simulink library "amg_high_precision_rtc"  (R2015b)
settings: Solver=ode45  StartTime=0.0  StopTime=10.0  RelTol=1e-3
libraries: simulink x207, waijung_soft_i2c_lib x11, amg_high_precision_rtc x10
(part 1 of 5)
settings Model: Creator=Krisada  LastModifiedBy=Aimagin
settings DataIOCC: SaveFormat=Array  SignalLoggingSaveFormat=ModelDataLogs
settings OptimizationCC: BlockReduction=off  DefaultParameterBehavior=Inlined  BufferReuse=off  ExpressionDepthLimit=2147483647
settings DebuggingCC: UnderspecifiedInitializationDetection=Classic  MergeDetectMultiDrivingBlocksExec=none  SolverPrmCheckMsg=warning  FcnCallInpInsideContextMsg=UseLocalSettings  StateNameClashWarn=warning  StrictBusMsg=Warning
settings HardwareCC: ProdBitPerPointer=32  ProdLargestAtomicFloat=None  ProdIntDivRoundTo=Undefined  ProdEndianess=Unspecified  ProdWordSize=32  ProdHWDeviceType=32-bit Generic
settings GRTTargetCC: CombineOutputUpdateFcns=off  GRTInterface=on
settings ConfigComp: CovModelRefEnable=Off

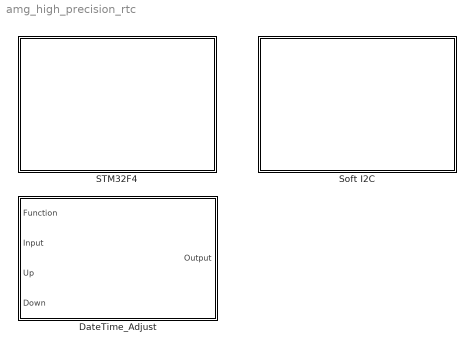
== system amg_high_precision_rtc ==
  DateTime_Adjust : Subsystem  TreatAsAtomicUnit=on  mask{state=0, max=99, min=0}
      mask prompts: state "Adjust state"; max "Max limit"; min "Min limit"
      settings: RTWFcnNameOpts=Use subsystem name  RTWFileNameOpts=Use function name
  STM32F4 : Subsystem
  Soft I2C : Subsystem

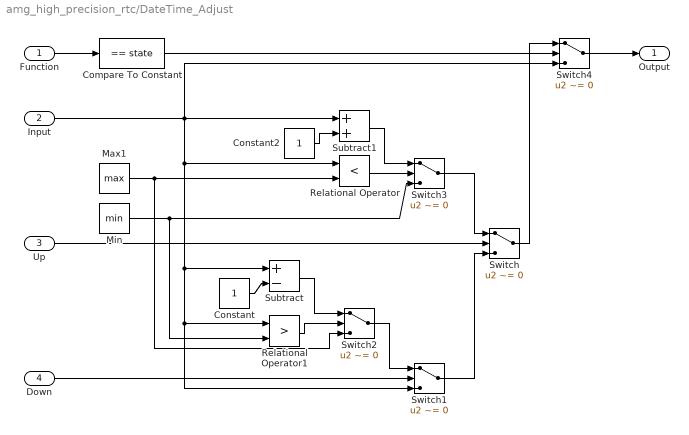
== system amg_high_precision_rtc/DateTime_Adjust ==
  Function : Inport
  Input : Inport  Port=2
  Up : Inport  Port=3
  Down : Inport  Port=4
  Compare To Constant : simulink/Logic and Bit Operations/Compare To Constant  SystemSampleTime=-1  relop===  const=state  LogicOutDataTypeMode=uint8  ZeroCross=off
  Constant : Constant  OutDataTypeStr=uint8
  Constant2 : Constant  OutDataTypeStr=uint8
  Max1 : Constant  Value=max  OutDataTypeStr=uint8
  Min : Constant  Value=min  OutDataTypeStr=uint8
  Relational Operator : RelationalOperator  Operator=<  OutDataTypeStr=boolean
  Relational Operator1 : RelationalOperator  Operator=>  OutDataTypeStr=boolean
  Subtract : Sum  Inputs=+-
  Subtract1 : Sum
  Switch{,1..4} (5 alike) : Switch  Criteria=u2 ~= 0
  Output : Outport
  wires:
  Switch1/1 -> Switch/3
  Input/1 -> Subtract/1, Switch1/3, Relational Operator1/1, Relational Operator/1, Subtract1/1, Switch4/3
  Relational Operator1/1 -> Switch2/2
  Subtract/1 -> Switch2/1
  Constant/1 -> Subtract/2
  Switch2/1 -> Switch1/1
  Relational Operator/1 -> Switch3/2
  Subtract1/1 -> Switch3/1
  Constant2/1 -> Subtract1/2
  Min/1 -> Switch3/3, Relational Operator1/2
  Max1/1 -> Relational Operator/2, Switch2/3
  Switch3/1 -> Switch/1
  Function/1 -> Compare To Constant/1
  Switch4/1 -> Output/1
  Compare To Constant/1 -> Switch4/2
  Switch/1 -> Switch4/1
  Down/1 -> Switch1/2
  Up/1 -> Switch/2

== system amg_high_precision_rtc/STM32F4 ==
  DS3231 Configure : Subsystem  mask(amg_high_precision_rtc){blockfunction=configure, module=1}
      mask prompts: blockfunction "Function"; module "I2C module"
      mask init:
      | amg_high_precision_rtc_callback('init');
      mask Help: web(fullfile(waijungdocroot,'DS3231_Configure.htm'), '-browser')
      mask TypeOptions blockfunction: temp | time | date | configure
      mask TypeOptions module: 1 | 2 | 3
      mask Callback module: amg_high_precision_rtc_callback('module');
      mask Display: text(0.5, 0.5, 'Port: I2C1','ver','middle','hor','center');port_label('input', 1,'SlvAddr');port_label('output', 1,'Status');port_label('input', 2,'(+) UP');port_label('input', 3,'(-) DOWN');port_label('input', 4,'(*) MODE');port_label('output', 2,'Enable');
  DS3231 Get Date : Subsystem  mask(amg_high_precision_rtc){blockfunction=date, module=1}
      mask prompts: blockfunction "Function"; module "I2C module"
      mask init:
      | amg_high_precision_rtc_callback('init');
      mask Help: web(fullfile(waijungdocroot,'DS3231_Get_Date.htm'), '-browser')
      mask TypeOptions blockfunction: temp | time | date
      mask TypeOptions module: 1 | 2 | 3
      mask Callback module: amg_high_precision_rtc_callback('module');
      mask Display: text(0.5, 0.5, 'Port: I2C1','ver','middle','hor','center');port_label('input', 1,'SlvAddr');port_label('output', 1,'Status');port_label('output', 2,'Day(1-7)');port_label('output', 3,'Date(1-31)');port_label('output', 4,'Month(1-12)');port_label('output', 5,'Year(0-99)');
  DS3231 Get Time : Subsystem  mask(amg_high_precision_rtc){blockfunction=time, module=1}
      mask prompts: blockfunction "Function"; module "I2C module"
      mask init:
      | amg_high_precision_rtc_callback('init');
      mask Help: web(fullfile(waijungdocroot,'DS3231_Get_Time.htm'), '-browser')
      mask TypeOptions blockfunction: temp | time | date
      mask TypeOptions module: 1 | 2 | 3
      mask Callback module: amg_high_precision_rtc_callback('module');
      mask Display: text(0.5, 0.5, 'Port: I2C1','ver','middle','hor','center');port_label('input', 1,'SlvAddr');port_label('output', 1,'Status');port_label('output', 2,'Hour(0-11/23)');port_label('output', 3,'Minute(0-59)');port_label('output', 4,'Second(0-59)');port_label('output', 5,'AM(0)/PM(1)');
  DS3231 Set Date : Subsystem  mask(amg_high_precision_rtc){blockfunction=setdate, module=1}
      mask prompts: blockfunction "Function"; module "I2C module"
      mask init:
      | amg_high_precision_rtc_callback('init');
      mask Help: web(fullfile(waijungdocroot,'DS3231_Get_Time.htm'), '-browser')
      mask TypeOptions blockfunction: setdate
      mask TypeOptions module: 1 | 2 | 3
      mask Callback module: amg_high_precision_rtc_callback('module');
      mask Display: text(0.5, 0.5, 'Port: I2C1','ver','middle','hor','center');port_label('input', 1,'SlvAddr');port_label('input', 2,'Date(1-31)');port_label('input', 3,'Month(1-12)');port_label('input', 4,'Year(0-99)');port_label('output', 1,'Status');
  DS3231 Set Time : Subsystem  mask(amg_high_precision_rtc){blockfunction=settime, module=1}
      mask prompts: blockfunction "Function"; module "I2C module"
      mask init:
      | amg_high_precision_rtc_callback('init');
      mask Help: web(fullfile(waijungdocroot,'DS3231_Get_Date.htm'), '-browser')
      mask TypeOptions blockfunction: settime
      mask TypeOptions module: 1 | 2 | 3
      mask Callback module: amg_high_precision_rtc_callback('module');
      mask Display: text(0.5, 0.5, 'Port: I2C1','ver','middle','hor','center');port_label('input', 1,'SlvAddr');port_label('input', 2,'Hour(0-11/23)');port_label('input', 3,'Minute(0-59)');port_label('input', 4,'Second(0-59)');port_label('output', 1,'Status');
  DS3231Temperture : Subsystem  mask(amg_high_precision_rtc){blockfunction=temp, module=1}
      mask prompts: blockfunction "Function"; module "I2C module"
      mask help:
      | The block implement temperature reading from DS3231 (Extremely Accurate RTC).
      | Its override the CONV bit, to force the temperature update, so the recommend sample time for this block is more than 0.5 seconds.
      | To get reading value from DS3231 device, this block generate 3 transaction of I2C as below:
      | 1. Read 2 bytes data from register 0x11 and 0x12 (Sequential read).
      | 2. Read 1 byte data from register 0x0F (Status) for poll BSY bit.
      | 3. Write 1 byte data to register 0x0E to force temperature conversion, CONV bit.
      mask init:
      | amg_high_precision_rtc_callback('init');
      mask Help: web(fullfile(waijungdocroot,'DS3231Temperture.htm'), '-browser')
      mask TypeOptions blockfunction: temp | time | date
      mask TypeOptions module: 1 | 2 | 3
      mask Callback module: amg_high_precision_rtc_callback('module');
      mask Display: text(0.5, 0.5, 'Port: I2C1','ver','middle','hor','center');port_label('input', 1,'SlvAddr');port_label('output', 1,'Status');port_label('output', 2,'Temp (C)');

== system amg_high_precision_rtc/Soft I2C ==
  Soft-DS3231 Configure : Subsystem  mask(amg_high_precision_rtc){blockfunction=configure, module=1}
      mask prompts: blockfunction "Function"; module "I2C module"
      mask init:
      | amg_high_precision_rtc_callback('init');
      mask Help: web(fullfile(waijungdocroot,'DS3231_Configure.htm'), '-browser')
      mask TypeOptions blockfunction: temp | time | date | configure
      mask TypeOptions module: 1 | 2 | 3 | 4 | 5 | 6 | 7 | 8 | 9 | 10 | 11 | 12 | 13 | 14 | 15 | 16 | 17 | 18 | 19 | 20 | 21 | 22 | 23 | 24 | 25 | 26 | 27 | 28 | 29 | 30 | 31 | 32
      mask Callback module: amg_high_precision_rtc_callback('module');
      mask Display: text(0.5, 0.5, 'Port: I2C1','ver','middle','hor','center');port_label('input', 1,'SlvAddr');port_label('output', 1,'Status');port_label('input', 2,'(+) UP');port_label('input', 3,'(-) DOWN');port_label('input', 4,'(*) MODE');port_label('output', 2,'Enable');
  Soft-DS3231 Get Date : Subsystem  mask(amg_high_precision_rtc){blockfunction=date, module=1}
      mask prompts: blockfunction "Function"; module "I2C module"
      mask init:
      | amg_high_precision_rtc_callback('init');
      mask Help: web(fullfile(waijungdocroot,'DS3231_Get_Date.htm'), '-browser')
      mask TypeOptions blockfunction: temp | time | date
      mask TypeOptions module: 1 | 2 | 3 | 4 | 5 | 6 | 7 | 8 | 9 | 10 | 11 | 12 | 13 | 14 | 15 | 16 | 17 | 18 | 19 | 20 | 21 | 22 | 23 | 24 | 25 | 26 | 27 | 28 | 29 | 30 | 31 | 32
      mask Callback module: amg_high_precision_rtc_callback('module');
      mask Display: text(0.5, 0.5, 'Port: I2C1','ver','middle','hor','center');port_label('input', 1,'SlvAddr');port_label('output', 1,'Status');port_label('output', 2,'Day(1-7)');port_label('output', 3,'Date(1-31)');port_label('output', 4,'Month(1-12)');port_label('output', 5,'Year(0-99)');
  Soft-DS3231 Get Time : Subsystem  mask(amg_high_precision_rtc){blockfunction=time, module=1}
      mask prompts: blockfunction "Function"; module "I2C module"
      mask init:
      | amg_high_precision_rtc_callback('init');
      mask Help: web(fullfile(waijungdocroot,'DS3231_Get_Time.htm'), '-browser')
      mask TypeOptions blockfunction: temp | time | date
      mask TypeOptions module: 1 | 2 | 3 | 4 | 5 | 6 | 7 | 8 | 9 | 10 | 11 | 12 | 13 | 14 | 15 | 16 | 17 | 18 | 19 | 20 | 21 | 22 | 23 | 24 | 25 | 26 | 27 | 28 | 29 | 30 | 31 | 32
      mask Callback module: amg_high_precision_rtc_callback('module');
      mask Display: text(0.5, 0.5, 'Port: I2C1','ver','middle','hor','center');port_label('input', 1,'SlvAddr');port_label('output', 1,'Status');port_label('output', 2,'Hour(0-11/23)');port_label('output', 3,'Minute(0-59)');port_label('output', 4,'Second(0-59)');port_label('output', 5,'AM(0)/PM(1)');
  Soft-DS3231 Set Date : Subsystem  mask(amg_high_precision_rtc){blockfunction=setdate, module=1}
      mask prompts: blockfunction "Function"; module "I2C module"
      mask init:
      | amg_high_precision_rtc_callback('init');
      mask Help: web(fullfile(waijungdocroot,'DS3231_Get_Time.htm'), '-browser')
      mask TypeOptions blockfunction: setdate
      mask TypeOptions module: 1 | 2 | 3 | 4 | 5 | 6 | 7 | 8 | 9 | 10 | 11 | 12 | 13 | 14 | 15 | 16 | 17 | 18 | 19 | 20 | 21 | 22 | 23 | 24 | 25 | 26 | 27 | 28 | 29 | 30 | 31 | 32
      mask Callback module: amg_high_precision_rtc_callback('module');
      mask Display: text(0.5, 0.5, 'Port: I2C1','ver','middle','hor','center');port_label('input', 1,'SlvAddr');port_label('input', 2,'Date(1-31)');port_label('input', 3,'Month(1-12)');port_label('input', 4,'Year(0-99)');port_label('output', 1,'Status');
  Soft-DS3231 Set Time : Subsystem  mask(amg_high_precision_rtc){blockfunction=settime, module=1}
      mask prompts: blockfunction "Function"; module "I2C module"
      mask init:
      | amg_high_precision_rtc_callback('init');
      mask Help: web(fullfile(waijungdocroot,'DS3231_Get_Date.htm'), '-browser')
      mask TypeOptions blockfunction: settime
      mask TypeOptions module: 1 | 2 | 3 | 4 | 5 | 6 | 7 | 8 | 9 | 10 | 11 | 12 | 13 | 14 | 15 | 16 | 17 | 18 | 19 | 20 | 21 | 22 | 23 | 24 | 25 | 26 | 27 | 28 | 29 | 30 | 31 | 32
      mask Callback module: amg_high_precision_rtc_callback('module');
      mask Display: text(0.5, 0.5, 'Port: I2C1','ver','middle','hor','center');port_label('input', 1,'SlvAddr');port_label('input', 2,'Hour(0-11/23)');port_label('input', 3,'Minute(0-59)');port_label('input', 4,'Second(0-59)');port_label('output', 1,'Status');
  Soft-DS3231Temperture : Subsystem  mask(amg_high_precision_rtc){blockfunction=temp, module=1}
      mask prompts: blockfunction "Function"; module "I2C module"
      mask help:
      | The block implement temperature reading from DS3231 (Extremely Accurate RTC).
      | Its override the CONV bit, to force the temperature update, so the recommend sample time for this block is more than 0.5 seconds.
      | To get reading value from DS3231 device, this block generate 3 transaction of I2C as below:
      | 1. Read 2 bytes data from register 0x11 and 0x12 (Sequential read).
      | 2. Read 1 byte data from register 0x0F (Status) for poll BSY bit.
      | 3. Write 1 byte data to register 0x0E to force temperature conversion, CONV bit.
      mask init:
      | amg_high_precision_rtc_callback('init');
      mask Help: web(fullfile(waijungdocroot,'DS3231Temperture.htm'), '-browser')
      mask TypeOptions blockfunction: temp | time | date
      mask TypeOptions module: 1 | 2 | 3 | 4 | 5 | 6 | 7 | 8 | 9 | 10 | 11 | 12 | 13 | 14 | 15 | 16 | 17 | 18 | 19 | 20 | 21 | 22 | 23 | 24 | 25 | 26 | 27 | 28 | 29 | 30 | 31 | 32
      mask Callback module: amg_high_precision_rtc_callback('module');
      mask Display: text(0.5, 0.5, 'Port: I2C1','ver','middle','hor','center');port_label('input', 1,'SlvAddr');port_label('output', 1,'Status');port_label('output', 2,'Temp (C)');

== system amg_high_precision_rtc/STM32F4/DS3231 Configure ==
  Slave Address : Inport
  Button UP : Inport  Port=2
  Button DOWN : Inport  Port=3
  Button MODE : Inport  Port=4
  Debouce4 : Subsystem  TreatAsAtomicUnit=on  mask{mode=Toggle Latch, prescale=256, debouce=255}
      mask prompts: prescale "Prescale (Debouce count)"; debouce "Debouce value"
      settings: RTWFcnNameOpts=Use subsystem name  RTWFileNameOpts=Use function name
      mask TypeOptions mode: Normal | Single Pulse | Toggle Latch
      mask Callback mode: waijung_intput_validation_callback('mode');
      mask TypeOptions prescale: 4 | 8 | 16 | 32 | 64 | 128 | 256 | 512 | 1024 | 2048 | 4096 | 8192
      mask Callback debouce: waijung_intput_validation_callback('prescale');
      mask Display: disp('Button Pressed\n(Toggle Latch)\nDebounce count: 256');
  Enabled Subsystem : Subsystem  TreatAsAtomicUnit=on
  Adjust state : Outport
  Adjust enable : Outport  Port=2
  wires:
  Slave Address/1 -> Enabled Subsystem/1(SlvAddr)
  Button UP/1 -> Enabled Subsystem/2(UP)
  Button DOWN/1 -> Enabled Subsystem/3(DOWN)
  Button MODE/1 -> Debouce4/1(In1), Enabled Subsystem/4(MODE)
  Debouce4/1(Out1) -> Enabled Subsystem/Enable, Adjust enable/1
  Enabled Subsystem/1(Adjust state) -> Adjust state/1

== system amg_high_precision_rtc/STM32F4/DS3231 Get Date ==
  Slave Address : Inport
  Compare To Zero : simulink/Logic and Bit Operations/Compare To Zero  SystemSampleTime=-1  relop===  LogicOutDataTypeMode=uint8  ZeroCross=off
  Convert : Subsystem  TreatAsAtomicUnit=on
  I2C Master Read/Write : S-Function  FunctionName=stm32f4_i2c  Parameters=configuration,module,transfer,clkspeed,timeout,sdapin,sclpin,writecount,readcount,inputtypearray,outputtypearray,confstr,sampletime,sampletimestr,blockid  SFunctionDeploymentMode=off  EnableBusSupport=off  mask(stm32f4_i2c){configuration=Transaction, module=1, lastmodule=3, transfer=Blocking, dutycycle=TLow/THigh = 2, clkspeed=400, timeout=25, writecount=1, readcount=4, sdapin=C9, sclpin=A8, waitwritetime=0, inputtypearray=[2 3 3], outputtypearray=[5 3 3 3 3 3], confstr=["C","9","A","8","1","1","6","0","I2C_DutyCycle_2","0"], sampletime=-1, sampletimestr=0, blockid=amg_high_precision_rtcDS3231GetDateI2CMasterReadWrite}
      mask prompts: module "I2C Module"; lastmodule "Last module"; transfer "Transfer mode"; dutycycle "Duty cycle in fast mode"; clkspeed "Clock speed (kHz)"; timeout "Timeout (ms)"; writecount "Bytes write count"; readcount "Bytes read count"; sdapin "SDA pin"; sclpin "SCL pin"; waitwritetime "Wait write time (ms), default is 0"; inputtypearray "Input type array"; outputtypearray "Output type array"; confstr "Configuration string"; sampletime "Sample time (sec)"; sampletimestr "Compiled sample time (sec) in string"
      mask init:
      | stm32f4_i2c_callback('init');
      mask Help: web(fullfile(waijungdocroot,'stm32f4_i2c_readwrite.htm'), '-browser')
      mask TypeOptions configuration: Setup | Transaction
      mask Callback configuration: stm32f4_i2c_callback('configuration');
      mask TypeOptions module: 1 | 2 | 3
      mask Callback module: stm32f4_i2c_callback('module');
      mask TypeOptions transfer: Blocking | Non-blocking
      mask TypeOptions dutycycle: TLow/THigh = 16/9 | TLow/THigh = 2
      mask Callback dutycycle: stm32f4_i2c_callback('dutycycle');
      mask Callback writecount: stm32f4_i2c_callback('writecount');
      mask Callback readcount: stm32f4_i2c_callback('readcount');
      mask TypeOptions sdapin: - | C9
      mask Callback sdapin: stm32f4_i2c_callback('sdapin');
      mask TypeOptions sclpin: - | A8
      mask Callback sclpin: stm32f4_i2c_callback('sclpin');
      mask Callback confstr: stm32f4_i2c_callback('confstr');
      mask Callback sampletime: stm32f4_i2c_callback('sampletime');
      mask Callback sampletimestr: stm32f4_i2c_callback('sampletimestr');
      mask Callback blockid: stm32f4_i2c_callback('blockid');
      mask Display: text(0.5, 0.5, 'Module: I2C1\nTransfer: Blocking\nWrite: 1 bytes\nRead: 4 bytes\nTs (sec): 0','ver','middle','hor','center');port_label('input', 1,'SlvAddr');port_label('input', 2,'Wr0 (uint8)');port_label('output', 1,'Status');port_label('output', 2,'Rd0 (uint8)');port_label('output', 3,'Rd1 (uint8)');port_label('output', 4,'Rd2 (uint8)');port_label('output', 5,'Rd3 (uint8)');
  REG_DATE : Constant  Value=hex2dec('03')  OutDataTypeStr=uint8
  Status : Outport
  Day : Outport  Port=2
  Date : Outport  Port=3
  Month : Outport  Port=4
  Year : Outport  Port=5
  wires:
  I2C Master Read/Write/4 -> Convert/3(In3)
  I2C Master Read/Write/3 -> Convert/2(In2)
  I2C Master Read/Write/2 -> Convert/1(In1)
  Compare To Zero/1 -> Status/1, Convert/Enable
  I2C Master Read/Write/1 -> Compare To Zero/1
  Slave Address/1 -> I2C Master Read/Write/1
  REG_DATE/1 -> I2C Master Read/Write/2
  I2C Master Read/Write/5 -> Convert/4(In4)
  Convert/1(Day) -> Day/1
  Convert/2(Date) -> Date/1
  Convert/4(Year) -> Year/1
  Convert/3(Month) -> Month/1

== system amg_high_precision_rtc/STM32F4/DS3231 Get Time ==
  Slave Address : Inport
  Compare To Zero : simulink/Logic and Bit Operations/Compare To Zero  SystemSampleTime=-1  relop===  LogicOutDataTypeMode=uint8  ZeroCross=off
  Convert : Subsystem  TreatAsAtomicUnit=on
  Data Type Conversion{,1..3} (4 alike) : DataTypeConversion  OutDataTypeStr=uint8
  I2C Master Read/Write : S-Function  FunctionName=stm32f4_i2c  Parameters=configuration,module,transfer,clkspeed,timeout,sdapin,sclpin,writecount,readcount,inputtypearray,outputtypearray,confstr,sampletime,sampletimestr,blockid  SFunctionDeploymentMode=off  EnableBusSupport=off  mask(stm32f4_i2c){configuration=Transaction, module=1, lastmodule=3, transfer=Blocking, dutycycle=TLow/THigh = 2, clkspeed=400, timeout=25, writecount=1, readcount=3, sdapin=C9, sclpin=A8, waitwritetime=0, inputtypearray=[2 3 3], outputtypearray=[4 3 3 3 3], confstr=["C","9","A","8","1","1","6","0","I2C_DutyCycle_2","0"], sampletime=-1, sampletimestr=0, blockid=amg_high_precision_rtcDS3231TimeI2CMasterReadWrite}
      mask prompts: module "I2C Module"; lastmodule "Last module"; transfer "Transfer mode"; dutycycle "Duty cycle in fast mode"; clkspeed "Clock speed (kHz)"; timeout "Timeout (ms)"; writecount "Bytes write count"; readcount "Bytes read count"; sdapin "SDA pin"; sclpin "SCL pin"; waitwritetime "Wait write time (ms), default is 0"; inputtypearray "Input type array"; outputtypearray "Output type array"; confstr "Configuration string"; sampletime "Sample time (sec)"; sampletimestr "Compiled sample time (sec) in string"
      mask init:
      | stm32f4_i2c_callback('init');
      mask Help: web(fullfile(waijungdocroot,'stm32f4_i2c_readwrite.htm'), '-browser')
      mask TypeOptions configuration: Setup | Transaction
      mask Callback configuration: stm32f4_i2c_callback('configuration');
      mask TypeOptions module: 1 | 2 | 3
      mask Callback module: stm32f4_i2c_callback('module');
      mask TypeOptions transfer: Blocking | Non-blocking
      mask TypeOptions dutycycle: TLow/THigh = 16/9 | TLow/THigh = 2
      mask Callback dutycycle: stm32f4_i2c_callback('dutycycle');
      mask Callback writecount: stm32f4_i2c_callback('writecount');
      mask Callback readcount: stm32f4_i2c_callback('readcount');
      mask TypeOptions sdapin: - | C9
      mask Callback sdapin: stm32f4_i2c_callback('sdapin');
      mask TypeOptions sclpin: - | A8
      mask Callback sclpin: stm32f4_i2c_callback('sclpin');
      mask Callback confstr: stm32f4_i2c_callback('confstr');
      mask Callback sampletime: stm32f4_i2c_callback('sampletime');
      mask Callback sampletimestr: stm32f4_i2c_callback('sampletimestr');
      mask Callback blockid: stm32f4_i2c_callback('blockid');
      mask Display: text(0.5, 0.5, 'Module: I2C1\nTransfer: Blocking\nWrite: 1 bytes\nRead: 3 bytes\nTs (sec): 0','ver','middle','hor','center');port_label('input', 1,'SlvAddr');port_label('input', 2,'Wr0 (uint8)');port_label('output', 1,'Status');port_label('output', 2,'Rd0 (uint8)');port_label('output', 3,'Rd1 (uint8)');port_label('output', 4,'Rd2 (uint8)');
  REG_TIME : Constant  Value=hex2dec('00')  OutDataTypeStr=uint8
  Status : Outport
  Hour : Outport  Port=2
  Minute : Outport  Port=3
  Second : Outport  Port=4
  AM/PM : Outport  Port=5
  wires:
  REG_TIME/1 -> I2C Master Read/Write/2
  Slave Address/1 -> I2C Master Read/Write/1
  I2C Master Read/Write/1 -> Compare To Zero/1
  Compare To Zero/1 -> Convert/Enable, Status/1
  I2C Master Read/Write/2 -> Convert/1(In1)
  I2C Master Read/Write/3 -> Convert/2(In2)
  I2C Master Read/Write/4 -> Convert/3(In3)
  Convert/3(Second) -> Data Type Conversion2/1
  Convert/2(Minute) -> Data Type Conversion1/1
  Convert/1(Hour) -> Data Type Conversion/1
  Convert/4(AM/PM) -> Data Type Conversion3/1
  Data Type Conversion/1 -> Hour/1
  Data Type Conversion1/1 -> Minute/1
  Data Type Conversion2/1 -> Second/1
  Data Type Conversion3/1 -> AM/PM/1

== system amg_high_precision_rtc/STM32F4/DS3231 Set Date ==
  SlvAddr : Inport
  Date : Inport  Port=2
  Month : Inport  Port=3
  Year : Inport  Port=4
  Constant : Constant  Value=4  OutDataTypeStr=uint8
  ConvertToBCD1 : Subsystem  TreatAsAtomicUnit=on
      settings: RTWFcnNameOpts=Use subsystem name  RTWFileNameOpts=Use function name
      mask Display: disp('Dec-to-BCD');
  ConvertToBCD2 : Subsystem  TreatAsAtomicUnit=on
      settings: RTWFcnNameOpts=Use subsystem name  RTWFileNameOpts=Use function name
      mask Display: disp('Dec-to-BCD');
  ConvertToBCD3 : Subsystem  TreatAsAtomicUnit=on
      settings: RTWFcnNameOpts=Use subsystem name  RTWFileNameOpts=Use function name
      mask Display: disp('Dec-to-BCD');
  I2C Master Read/Write : S-Function  FunctionName=stm32f4_i2c  Parameters=configuration,module,transfer,clkspeed,timeout,sdapin,sclpin,writecount,readcount,inputtypearray,outputtypearray,confstr,sampletime,sampletimestr,blockid  SFunctionDeploymentMode=off  EnableBusSupport=off  mask(stm32f4_i2c){configuration=Transaction, module=1, lastmodule=3, transfer=Blocking, dutycycle=TLow/THigh = 2, clkspeed=400, timeout=25, writecount=4, readcount=0, sdapin=C9, sclpin=A8, waitwritetime=0, inputtypearray=[5 3 3 3 3 3], outputtypearray=[1 3], confstr=["C","9","A","8","1","1","6","0","I2C_DutyCycle_2","0"], sampletime=-1, sampletimestr=0, blockid=DS3231SetDateI2CMasterReadWrite}
      mask prompts: module "I2C Module"; lastmodule "Last module"; transfer "Transfer mode"; dutycycle "Duty cycle in fast mode"; clkspeed "Clock speed (kHz)"; timeout "Timeout (ms)"; writecount "Bytes write count"; readcount "Bytes read count"; sdapin "SDA pin"; sclpin "SCL pin"; waitwritetime "Wait write time (ms), default is 0"; inputtypearray "Input type array"; outputtypearray "Output type array"; confstr "Configuration string"; sampletime "Sample time (sec)"; sampletimestr "Compiled sample time (sec) in string"
      mask init:
      | stm32f4_i2c_callback('init');
      mask Help: web(fullfile(waijungdocroot,'stm32f4_i2c_readwrite.htm'), '-browser')
      mask TypeOptions configuration: Setup | Transaction
      mask Callback configuration: stm32f4_i2c_callback('configuration');
      mask TypeOptions module: 1 | 2 | 3
      mask Callback module: stm32f4_i2c_callback('module');
      mask TypeOptions transfer: Blocking | Non-blocking
      mask TypeOptions dutycycle: TLow/THigh = 16/9 | TLow/THigh = 2
      mask Callback dutycycle: stm32f4_i2c_callback('dutycycle');
      mask Callback writecount: stm32f4_i2c_callback('writecount');
      mask Callback readcount: stm32f4_i2c_callback('readcount');
      mask TypeOptions sdapin: - | C9
      mask Callback sdapin: stm32f4_i2c_callback('sdapin');
      mask TypeOptions sclpin: - | A8
      mask Callback sclpin: stm32f4_i2c_callback('sclpin');
      mask Callback confstr: stm32f4_i2c_callback('confstr');
      mask Callback sampletime: stm32f4_i2c_callback('sampletime');
      mask Callback sampletimestr: stm32f4_i2c_callback('sampletimestr');
      mask Callback blockid: stm32f4_i2c_callback('blockid');
      mask Display: text(0.5, 0.5, 'Module: I2C1\nTransfer: Blocking\nWrite: 4 bytes\nRead: 0 bytes\nTs (sec): 0','ver','middle','hor','center');port_label('input', 1,'SlvAddr');port_label('input', 2,'Wr0 (uint8)');port_label('input', 3,'Wr1 (uint8)');port_label('input', 4,'Wr2 (uint8)');port_label('input', 5,'Wr3 (uint8)');port_label('output', 1,'Status');
  Out1 : Outport
  wires:
  SlvAddr/1 -> I2C Master Read/Write/1
  Constant/1 -> I2C Master Read/Write/2
  I2C Master Read/Write/1 -> Out1/1
  ConvertToBCD2/1(Out1) -> I2C Master Read/Write/3
  ConvertToBCD1/1(Out1) -> I2C Master Read/Write/4
  ConvertToBCD3/1(Out1) -> I2C Master Read/Write/5
  Date/1 -> ConvertToBCD2/1(In1)
  Month/1 -> ConvertToBCD1/1(In1)
  Year/1 -> ConvertToBCD3/1(In1)

== system amg_high_precision_rtc/STM32F4/DS3231 Set Time ==
  SlvAddr : Inport
  Hour : Inport  Port=2
  Minute : Inport  Port=3
  Second : Inport  Port=4
  Constant1 : Constant  Value=0  OutDataTypeStr=uint8
  ConvertToBCD1 : Subsystem  TreatAsAtomicUnit=on
      settings: RTWFcnNameOpts=Use subsystem name  RTWFileNameOpts=Use function name
      mask Display: disp('Dec-to-BCD');
  ConvertToBCD2 : Subsystem  TreatAsAtomicUnit=on
      settings: RTWFcnNameOpts=Use subsystem name  RTWFileNameOpts=Use function name
      mask Display: disp('Dec-to-BCD');
  ConvertToBCD3 : Subsystem  TreatAsAtomicUnit=on
      settings: RTWFcnNameOpts=Use subsystem name  RTWFileNameOpts=Use function name
      mask Display: disp('Dec-to-BCD');
  I2C Master Read/Write1 : S-Function  FunctionName=stm32f4_i2c  Parameters=configuration,module,transfer,clkspeed,timeout,sdapin,sclpin,writecount,readcount,inputtypearray,outputtypearray,confstr,sampletime,sampletimestr,blockid  SFunctionDeploymentMode=off  EnableBusSupport=off  mask(stm32f4_i2c){configuration=Transaction, module=1, lastmodule=3, transfer=Blocking, dutycycle=TLow/THigh = 2, clkspeed=400, timeout=25, writecount=4, readcount=0, sdapin=C9, sclpin=A8, waitwritetime=0, inputtypearray=[5 3 3 3 3 3], outputtypearray=[1 3], confstr=["C","9","A","8","1","1","6","0","I2C_DutyCycle_2","0"], sampletime=-1, sampletimestr=0.01, blockid=configureDS3231ConfigureEnabledSubsystemSubsystemEnabledSubsystemI2CMasterReadWrite1}
      mask prompts: module "I2C Module"; lastmodule "Last module"; transfer "Transfer mode"; dutycycle "Duty cycle in fast mode"; clkspeed "Clock speed (kHz)"; timeout "Timeout (ms)"; writecount "Bytes write count"; readcount "Bytes read count"; sdapin "SDA pin"; sclpin "SCL pin"; waitwritetime "Wait write time (ms), default is 0"; inputtypearray "Input type array"; outputtypearray "Output type array"; confstr "Configuration string"; sampletime "Sample time (sec)"; sampletimestr "Compiled sample time (sec) in string"
      mask init:
      | stm32f4_i2c_callback('init');
      mask Help: web(fullfile(waijungdocroot,'stm32f4_i2c_readwrite.htm'), '-browser')
      mask TypeOptions configuration: Setup | Transaction
      mask Callback configuration: stm32f4_i2c_callback('configuration');
      mask TypeOptions module: 1 | 2 | 3
      mask Callback module: stm32f4_i2c_callback('module');
      mask TypeOptions transfer: Blocking | Non-blocking
      mask TypeOptions dutycycle: TLow/THigh = 16/9 | TLow/THigh = 2
      mask Callback dutycycle: stm32f4_i2c_callback('dutycycle');
      mask Callback writecount: stm32f4_i2c_callback('writecount');
      mask Callback readcount: stm32f4_i2c_callback('readcount');
      mask TypeOptions sdapin: - | C9
      mask Callback sdapin: stm32f4_i2c_callback('sdapin');
      mask TypeOptions sclpin: - | A8
      mask Callback sclpin: stm32f4_i2c_callback('sclpin');
      mask Callback confstr: stm32f4_i2c_callback('confstr');
      mask Callback sampletime: stm32f4_i2c_callback('sampletime');
      mask Callback sampletimestr: stm32f4_i2c_callback('sampletimestr');
      mask Callback blockid: stm32f4_i2c_callback('blockid');
      mask Display: text(0.5, 0.5, 'Module: I2C1\nTransfer: Blocking\nWrite: 4 bytes\nRead: 0 bytes\nTs (sec): 0.01','ver','middle','hor','center');port_label('input', 1,'SlvAddr');port_label('input', 2,'Wr0 (uint8)');port_label('input', 3,'Wr1 (uint8)');port_label('input', 4,'Wr2 (uint8)');port_label('input', 5,'Wr3 (uint8)');port_label('output', 1,'Status');
  Out1 : Outport
  wires:
  ConvertToBCD3/1(Out1) -> I2C Master Read/Write1/3
  ConvertToBCD2/1(Out1) -> I2C Master Read/Write1/5
  ConvertToBCD1/1(Out1) -> I2C Master Read/Write1/4
  I2C Master Read/Write1/1 -> Out1/1
  Constant1/1 -> I2C Master Read/Write1/2
  SlvAddr/1 -> I2C Master Read/Write1/1
  Hour/1 -> ConvertToBCD2/1(In1)
  Minute/1 -> ConvertToBCD1/1(In1)
  Second/1 -> ConvertToBCD3/1(In1)

== system amg_high_precision_rtc/STM32F4/DS3231Temperture ==
  Slave Address : Inport
  Check Busy/ Write Conv : Subsystem
  Compare To Zero : simulink/Logic and Bit Operations/Compare To Zero  SystemSampleTime=-1  relop===  LogicOutDataTypeMode=uint8  ZeroCross=off
  Convert : Subsystem  TreatAsAtomicUnit=on
  I2C Master Read/Write : S-Function  FunctionName=stm32f4_i2c  Parameters=configuration,module,transfer,clkspeed,timeout,sdapin,sclpin,writecount,readcount,inputtypearray,outputtypearray,confstr,sampletime,sampletimestr,blockid  SFunctionDeploymentMode=off  EnableBusSupport=off  mask(stm32f4_i2c){configuration=Transaction, module=1, lastmodule=3, transfer=Blocking, dutycycle=TLow/THigh = 2, clkspeed=400, timeout=25, writecount=1, readcount=2, sdapin=C9, sclpin=A8, waitwritetime=0, inputtypearray=[2 3 3], outputtypearray=[3 3 3 3], confstr=["C","9","A","8","1","3","4","2","I2C_DutyCycle_2","0"], sampletime=-1, sampletimestr=0, blockid=amg_high_precision_rtcTempertureReadI2CMasterReadWrite}
      mask prompts: module "I2C Module"; lastmodule "Last module"; transfer "Transfer mode"; dutycycle "Duty cycle in fast mode"; clkspeed "Clock speed (kHz)"; timeout "Timeout (ms)"; writecount "Bytes write count"; readcount "Bytes read count"; sdapin "SDA pin"; sclpin "SCL pin"; waitwritetime "Wait write time (ms), default is 0"; inputtypearray "Input type array"; outputtypearray "Output type array"; confstr "Configuration string"; sampletime "Sample time (sec)"; sampletimestr "Compiled sample time (sec) in string"
      mask init:
      | stm32f4_i2c_callback('init');
      mask Help: web(fullfile(waijungdocroot,'stm32f4_i2c_readwrite.htm'), '-browser')
      mask TypeOptions configuration: Setup | Transaction
      mask Callback configuration: stm32f4_i2c_callback('configuration');
      mask TypeOptions module: 1 | 2 | 3
      mask Callback module: stm32f4_i2c_callback('module');
      mask TypeOptions transfer: Blocking | Non-blocking
      mask TypeOptions dutycycle: TLow/THigh = 16/9 | TLow/THigh = 2
      mask Callback dutycycle: stm32f4_i2c_callback('dutycycle');
      mask Callback writecount: stm32f4_i2c_callback('writecount');
      mask Callback readcount: stm32f4_i2c_callback('readcount');
      mask TypeOptions sdapin: - | C9
      mask Callback sdapin: stm32f4_i2c_callback('sdapin');
      mask TypeOptions sclpin: - | A8
      mask Callback sclpin: stm32f4_i2c_callback('sclpin');
      mask Callback confstr: stm32f4_i2c_callback('confstr');
      mask Callback sampletime: stm32f4_i2c_callback('sampletime');
      mask Callback sampletimestr: stm32f4_i2c_callback('sampletimestr');
      mask Callback blockid: stm32f4_i2c_callback('blockid');
      mask Display: text(0.5, 0.5, 'Module: I2C1\nTransfer: Blocking\nWrite: 1 bytes\nRead: 2 bytes\nTs (sec): 0','ver','middle','hor','center');port_label('input', 1,'SlvAddr');port_label('input', 2,'Wr0 (uint8)');port_label('output', 1,'Status');port_label('output', 2,'Rd0 (uint8)');port_label('output', 3,'Rd1 (uint8)');
  REG_TEMP : Constant  Value=hex2dec('11')  OutDataTypeStr=uint8
  Status : Outport
  Temperature (C) : Outport  Port=2
  wires:
  Slave Address/1 -> I2C Master Read/Write/1, Check Busy/ Write Conv/1(In1)
  REG_TEMP/1 -> I2C Master Read/Write/2
  I2C Master Read/Write/1 -> Status/1, Compare To Zero/1
  Compare To Zero/1 -> Convert/Enable, Check Busy/ Write Conv/Enable
  I2C Master Read/Write/2 -> Convert/1(In1)
  I2C Master Read/Write/3 -> Convert/2(In2)
  Convert/1(Reading) -> Temperature (C)/1

== system amg_high_precision_rtc/Soft I2C/Soft-DS3231 Configure ==
  Slave Address : Inport
  Button UP : Inport  Port=2
  Button DOWN : Inport  Port=3
  Button MODE : Inport  Port=4
  Debouce4 : Subsystem  TreatAsAtomicUnit=on  mask{mode=Toggle Latch, prescale=256, debouce=255}
      mask prompts: prescale "Prescale (Debouce count)"; debouce "Debouce value"
      settings: RTWFcnNameOpts=Use subsystem name  RTWFileNameOpts=Use function name
      mask TypeOptions mode: Normal | Single Pulse | Toggle Latch
      mask Callback mode: waijung_intput_validation_callback('mode');
      mask TypeOptions prescale: 4 | 8 | 16 | 32 | 64 | 128 | 256 | 512 | 1024 | 2048 | 4096 | 8192
      mask Callback debouce: waijung_intput_validation_callback('prescale');
      mask Display: disp('Button Pressed\n(Toggle Latch)\nDebounce count: 256');
  Enabled Subsystem : Subsystem  TreatAsAtomicUnit=on
  Adjust state : Outport
  Adjust enable : Outport  Port=2
  wires:
  Enabled Subsystem/1(Adjust state) -> Adjust state/1
  Debouce4/1(Out1) -> Adjust enable/1, Enabled Subsystem/Enable
  Button MODE/1 -> Enabled Subsystem/4(MODE), Debouce4/1(In1)
  Button DOWN/1 -> Enabled Subsystem/3(DOWN)
  Button UP/1 -> Enabled Subsystem/2(UP)
  Slave Address/1 -> Enabled Subsystem/1(SlvAddr)

== system amg_high_precision_rtc/Soft I2C/Soft-DS3231 Get Date ==
  Slave Address : Inport
  Compare To Zero : simulink/Logic and Bit Operations/Compare To Zero  SystemSampleTime=-1  relop===  LogicOutDataTypeMode=uint8  ZeroCross=off
  Convert : Subsystem  TreatAsAtomicUnit=on
  REG_DATE : Constant  Value=hex2dec('03')  OutDataTypeStr=uint8
  Soft I2C Master Read/Write : waijung_soft_i2c_lib/Soft I2C Master Read//Write  conf=ReadWrite  targetname=0  module=1  transfer=Blocking  clk=100  timeout=25  sdapins={'A4','A6'}  sclpins='A5'  writecount=1  readcount=4  waittime=0  forcestop=off  portpinstr=0  sampletime=-1  blockid=SoftI2CSoftDS3231GetDateSoftI2CMasterReadWrite  inputporttype=[3 3]  inputportwidth=[]  inputportlabel={'SlvAddr' 'Wr0 (uint8)'}  outputporttype="[3 3 3 3 3    ]"  outputportwidth=[1 1 1 1 1]  outputportlabel={'Status' 'Rd0 (uint8)' 'Rd1 (uint8)' 'Rd2 (uint8)' 'Rd3 (uint8)'}  compat=0  optionstring=[]
  Status : Outport
  Day : Outport  Port=2
  Date : Outport  Port=3
  Month : Outport  Port=4
  Year : Outport  Port=5
  wires:
  Convert/3(Month) -> Month/1
  Convert/4(Year) -> Year/1
  Convert/2(Date) -> Date/1
  Convert/1(Day) -> Day/1
  Soft I2C Master Read/Write/5 -> Convert/4(In4)
  REG_DATE/1 -> Soft I2C Master Read/Write/2
  Slave Address/1 -> Soft I2C Master Read/Write/1
  Soft I2C Master Read/Write/1 -> Compare To Zero/1
  Compare To Zero/1 -> Convert/Enable, Status/1
  Soft I2C Master Read/Write/2 -> Convert/1(In1)
  Soft I2C Master Read/Write/3 -> Convert/2(In2)
  Soft I2C Master Read/Write/4 -> Convert/3(In3)

== system amg_high_precision_rtc/Soft I2C/Soft-DS3231 Get Time ==
  Slave Address : Inport
  Compare To Zero : simulink/Logic and Bit Operations/Compare To Zero  SystemSampleTime=-1  relop===  LogicOutDataTypeMode=uint8  ZeroCross=off
  Convert : Subsystem  TreatAsAtomicUnit=on
  Data Type Conversion{,1..3} (4 alike) : DataTypeConversion  OutDataTypeStr=uint8
  REG_TIME : Constant  Value=hex2dec('00')  OutDataTypeStr=uint8
  Soft I2C Master Read/Write : waijung_soft_i2c_lib/Soft I2C Master Read//Write  conf=ReadWrite  targetname=0  module=1  transfer=Blocking  clk=100  timeout=25  sdapins={'A4','A6'}  sclpins='A5'  writecount=1  readcount=3  waittime=0  forcestop=off  portpinstr=0  sampletime=-1  blockid=SoftI2CSoftDS3231GetTimeSoftI2CMasterReadWrite  inputporttype=[3 3]  inputportwidth=[]  inputportlabel={'SlvAddr' 'Wr0 (uint8)'}  outputporttype="[3 3 3 3   ]"  outputportwidth=[1 1 1 1]  outputportlabel={'Status' 'Rd0 (uint8)' 'Rd1 (uint8)' 'Rd2 (uint8)'}  compat=0  optionstring=[]
  Status : Outport
  Hour : Outport  Port=2
  Minute : Outport  Port=3
  Second : Outport  Port=4
  AM/PM : Outport  Port=5
  wires:
  Data Type Conversion3/1 -> AM/PM/1
  Data Type Conversion2/1 -> Second/1
  Data Type Conversion1/1 -> Minute/1
  Data Type Conversion/1 -> Hour/1
  Convert/4(AM/PM) -> Data Type Conversion3/1
  Convert/1(Hour) -> Data Type Conversion/1
  Convert/2(Minute) -> Data Type Conversion1/1
  Convert/3(Second) -> Data Type Conversion2/1
  Soft I2C Master Read/Write/4 -> Convert/3(In3)
  Soft I2C Master Read/Write/3 -> Convert/2(In2)
  Soft I2C Master Read/Write/2 -> Convert/1(In1)
  Compare To Zero/1 -> Status/1, Convert/Enable
  Soft I2C Master Read/Write/1 -> Compare To Zero/1
  Slave Address/1 -> Soft I2C Master Read/Write/1
  REG_TIME/1 -> Soft I2C Master Read/Write/2

== system amg_high_precision_rtc/Soft I2C/Soft-DS3231 Set Date ==
  SlvAddr : Inport
  Date : Inport  Port=2
  Month : Inport  Port=3
  Year : Inport  Port=4
  Constant : Constant  Value=4  OutDataTypeStr=uint8
  ConvertToBCD1 : Subsystem  TreatAsAtomicUnit=on
      settings: RTWFcnNameOpts=Use subsystem name  RTWFileNameOpts=Use function name
      mask Display: disp('Dec-to-BCD');
  ConvertToBCD2 : Subsystem  TreatAsAtomicUnit=on
      settings: RTWFcnNameOpts=Use subsystem name  RTWFileNameOpts=Use function name
      mask Display: disp('Dec-to-BCD');
  ConvertToBCD3 : Subsystem  TreatAsAtomicUnit=on
      settings: RTWFcnNameOpts=Use subsystem name  RTWFileNameOpts=Use function name
      mask Display: disp('Dec-to-BCD');
  Soft I2C Master Read/Write : waijung_soft_i2c_lib/Soft I2C Master Read//Write  conf=ReadWrite  targetname=0  module=1  transfer=Blocking  clk=100  timeout=25  sdapins={'A4','A6'}  sclpins='A5'  writecount=4  readcount=0  waittime=0  forcestop=off  portpinstr=0  sampletime=-1  blockid=SoftI2CSoftDS3231SetDateSoftI2CMasterReadWrite  inputporttype=[3 3 3 3 3]  inputportwidth=[]  inputportlabel={'SlvAddr' 'Wr0 (uint8)' 'Wr1 (uint8)' 'Wr2 (uint8)' 'Wr3 (uint8)'}  outputporttype=[3]  outputportwidth=[1]  outputportlabel={'Status'}  compat=0  optionstring=[]
  Out1 : Outport
  wires:
  Year/1 -> ConvertToBCD3/1(In1)
  Month/1 -> ConvertToBCD1/1(In1)
  Date/1 -> ConvertToBCD2/1(In1)
  ConvertToBCD3/1(Out1) -> Soft I2C Master Read/Write/5
  ConvertToBCD1/1(Out1) -> Soft I2C Master Read/Write/4
  ConvertToBCD2/1(Out1) -> Soft I2C Master Read/Write/3
  Soft I2C Master Read/Write/1 -> Out1/1
  Constant/1 -> Soft I2C Master Read/Write/2
  SlvAddr/1 -> Soft I2C Master Read/Write/1

== system amg_high_precision_rtc/Soft I2C/Soft-DS3231 Set Time ==
  SlvAddr : Inport
  Hour : Inport  Port=2
  Minute : Inport  Port=3
  Second : Inport  Port=4
  Constant1 : Constant  Value=0  OutDataTypeStr=uint8
  ConvertToBCD1 : Subsystem  TreatAsAtomicUnit=on
      settings: RTWFcnNameOpts=Use subsystem name  RTWFileNameOpts=Use function name
      mask Display: disp('Dec-to-BCD');
  ConvertToBCD2 : Subsystem  TreatAsAtomicUnit=on
      settings: RTWFcnNameOpts=Use subsystem name  RTWFileNameOpts=Use function name
      mask Display: disp('Dec-to-BCD');
  ConvertToBCD3 : Subsystem  TreatAsAtomicUnit=on
      settings: RTWFcnNameOpts=Use subsystem name  RTWFileNameOpts=Use function name
      mask Display: disp('Dec-to-BCD');
  Soft I2C Master Read/Write : waijung_soft_i2c_lib/Soft I2C Master Read//Write  conf=ReadWrite  targetname=0  module=1  transfer=Blocking  clk=100  timeout=25  sdapins={'A4','A6'}  sclpins='A5'  writecount=4  readcount=0  waittime=0  forcestop=off  portpinstr=0  sampletime=inf  blockid=SoftI2CSoftDS3231SetTimeSoftI2CMasterReadWrite  inputporttype=[3 3 3 3 3]  inputportwidth=[]  inputportlabel={'SlvAddr' 'Wr0 (uint8)' 'Wr1 (uint8)' 'Wr2 (uint8)' 'Wr3 (uint8)'}  outputporttype=[3]  outputportwidth=[1]  outputportlabel={'Status'}  compat=0  optionstring=[]
  Out1 : Outport
  wires:
  Second/1 -> ConvertToBCD3/1(In1)
  Minute/1 -> ConvertToBCD1/1(In1)
  Hour/1 -> ConvertToBCD2/1(In1)
  SlvAddr/1 -> Soft I2C Master Read/Write/1
  Constant1/1 -> Soft I2C Master Read/Write/2
  ConvertToBCD1/1(Out1) -> Soft I2C Master Read/Write/4
  ConvertToBCD2/1(Out1) -> Soft I2C Master Read/Write/5
  ConvertToBCD3/1(Out1) -> Soft I2C Master Read/Write/3
  Soft I2C Master Read/Write/1 -> Out1/1

== system amg_high_precision_rtc/Soft I2C/Soft-DS3231Temperture ==
  Slave Address : Inport
  Check Busy/ Write Conv : Subsystem
  Compare To Zero : simulink/Logic and Bit Operations/Compare To Zero  SystemSampleTime=-1  relop===  LogicOutDataTypeMode=uint8  ZeroCross=off
  Convert : Subsystem  TreatAsAtomicUnit=on
  REG_TEMP : Constant  Value=hex2dec('11')  OutDataTypeStr=uint8
  Soft I2C Master Read/Write : waijung_soft_i2c_lib/Soft I2C Master Read//Write  conf=ReadWrite  targetname=0  module=1  transfer=Blocking  clk=100  timeout=25  sdapins={'A4','A6'}  sclpins='A5'  writecount=1  readcount=2  waittime=0  forcestop=off  portpinstr=0  sampletime=-1  blockid=SoftI2CSoftDS3231TempertureSoftI2CMasterReadWrite  inputporttype=[3 3]  inputportwidth=[]  inputportlabel={'SlvAddr' 'Wr0 (uint8)'}  outputporttype="[3 3 3  ]"  outputportwidth=[1 1 1]  outputportlabel={'Status' 'Rd0 (uint8)' 'Rd1 (uint8)'}  compat=0  optionstring=[]
  Status : Outport
  Temperature (C) : Outport  Port=2
  wires:
  Convert/1(Reading) -> Temperature (C)/1
  Soft I2C Master Read/Write/3 -> Convert/2(In2)
  Soft I2C Master Read/Write/2 -> Convert/1(In1)
  Compare To Zero/1 -> Check Busy/ Write Conv/Enable, Convert/Enable
  Soft I2C Master Read/Write/1 -> Compare To Zero/1, Status/1
  REG_TEMP/1 -> Soft I2C Master Read/Write/2
  Slave Address/1 -> Check Busy/ Write Conv/1(In1), Soft I2C Master Read/Write/1

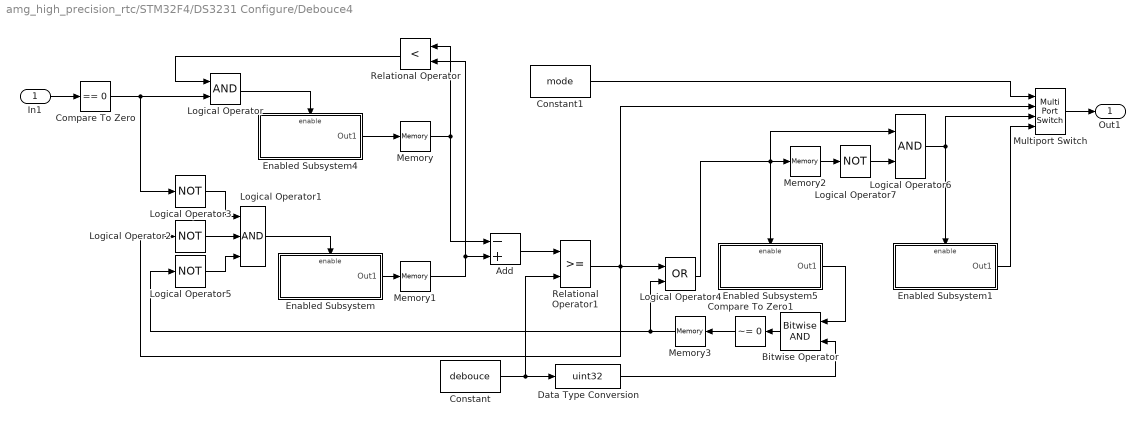
== system amg_high_precision_rtc/STM32F4/DS3231 Configure/Debouce4 ==
  In1 : Inport
  Add : Sum  Inputs=-+  OutDataTypeStr=int32
  Bitwise Operator : simulink/Logic and Bit Operations/Bitwise Operator  logicop=AND  UseBitMask=off  NumInputPorts=2  BitMask=debouce  BitMaskRealWorld=Stored Integer
  Compare To Zero : simulink/Logic and Bit Operations/Compare To Zero  SystemSampleTime=-1  relop===  LogicOutDataTypeMode=uint8  ZeroCross=off
  Compare To Zero1 : simulink/Logic and Bit Operations/Compare To Zero  SystemSampleTime=-1  relop=~=  LogicOutDataTypeMode=boolean  ZeroCross=off
  Constant : Constant  Value=debouce  OutDataTypeStr=int32
  Constant1 : Constant  Value=mode  OutDataTypeStr=int32
  Data Type Conversion : DataTypeConversion  OutDataTypeStr=uint32
  Enabled Subsystem : Subsystem  TreatAsAtomicUnit=on
  Enabled Subsystem1 : Subsystem  TreatAsAtomicUnit=on
  Enabled Subsystem4 : Subsystem  TreatAsAtomicUnit=on
  Enabled Subsystem5 : Subsystem  TreatAsAtomicUnit=on
  Logical Operator : Logic  AllPortsSameDT=off  OutDataTypeStr=boolean
  Logical Operator1 : Logic  Inputs=3  AllPortsSameDT=off  OutDataTypeStr=boolean
  Logical Operator{2..3,5,7} (4 alike) : Logic  Operator=NOT  AllPortsSameDT=off  OutDataTypeStr=boolean
  Logical Operator4 : Logic  Operator=OR  AllPortsSameDT=off  OutDataTypeStr=boolean
  Logical Operator6 : Logic  AllPortsSameDT=off  OutDataTypeStr=boolean
  Memory{,1..3} (4 alike) : Memory  LinearizeMemory=on
  Multiport Switch : MultiPortSwitch
  Relational Operator : RelationalOperator  Operator=<  OutDataTypeStr=boolean
  Relational Operator1 : RelationalOperator  OutDataTypeStr=boolean  InputSameDT=on
  Out1 : Outport
  wires:
  Constant1/1 -> Multiport Switch/1
  Multiport Switch/1 -> Out1/1
  Data Type Conversion/1 -> Bitwise Operator/2
  Enabled Subsystem1/1(Out1) -> Multiport Switch/4
  Logical Operator6/1 -> Enabled Subsystem1/Enable, Multiport Switch/3
  In1/1 -> Compare To Zero/1
  Enabled Subsystem/1(Out1) -> Memory1/1
  Enabled Subsystem4/1(Out1) -> Memory/1
  Memory/1 -> Relational Operator/1, Add/1
  Memory1/1 -> Add/2, Relational Operator/2
  Compare To Zero/1 -> Logical Operator/2, Logical Operator3/1
  Logical Operator/1 -> Enabled Subsystem4/Enable
  Relational Operator/1 -> Logical Operator/1
  Add/1 -> Relational Operator1/1
  Constant/1 -> Data Type Conversion/1, Relational Operator1/2
  Logical Operator2/1 -> Logical Operator1/2
  Memory3/1 -> Logical Operator4/2, Logical Operator5/1
  Logical Operator5/1 -> Logical Operator1/3
  Logical Operator3/1 -> Logical Operator1/1
  Compare To Zero1/1 -> Memory3/1
  Bitwise Operator/1 -> Compare To Zero1/1
  Enabled Subsystem5/1(Out1) -> Bitwise Operator/1
  Logical Operator4/1 -> Enabled Subsystem5/Enable, Memory2/1, Logical Operator6/1
  Memory2/1 -> Logical Operator7/1
  Logical Operator7/1 -> Logical Operator6/2
  Relational Operator1/1 -> Multiport Switch/2, Logical Operator4/1, Logical Operator2/1
  Logical Operator1/1 -> Enabled Subsystem/Enable

== system amg_high_precision_rtc/STM32F4/DS3231 Configure/Enabled Subsystem ==
  note: # Mode ID
      | 0 - DD
      | 1 - MM
      | 2 - YY
      | 3 - HH
      | 4 - MM
      | 5 - SS
  SlvAddr : Inport
  UP : Inport  Port=2
  DOWN : Inport  Port=3
  MODE : Inport  Port=4
  Enable : EnablePort  PropagateVarSize=During execution
  Debouce1 : Subsystem  TreatAsAtomicUnit=on  mask{mode=Single Pulse, prescale=4, debouce=7}
      mask prompts: prescale "Prescale (Debouce count)"; debouce "Debouce value"
      settings: RTWFcnNameOpts=Use subsystem name  RTWFileNameOpts=Use function name
      mask TypeOptions mode: Normal | Single Pulse | Toggle Latch
      mask Callback mode: waijung_intput_validation_callback('mode');
      mask TypeOptions prescale: 4 | 8 | 16 | 32 | 64 | 128 | 256 | 512 | 1024 | 2048 | 4096 | 8192
      mask Callback debouce: waijung_intput_validation_callback('prescale');
      mask Display: disp('Button Pressed\n(Normal)');
  Debouce2 : Subsystem  TreatAsAtomicUnit=on  mask{mode=Single Pulse, prescale=4, debouce=3}
      mask prompts: prescale "Prescale (Debouce count)"; debouce "Debouce value"
      settings: RTWFcnNameOpts=Use subsystem name  RTWFileNameOpts=Use function name
      mask TypeOptions mode: Normal | Single Pulse | Toggle Latch
      mask Callback mode: waijung_intput_validation_callback('mode');
      mask TypeOptions prescale: 4 | 8 | 16 | 32 | 64 | 128 | 256 | 512 | 1024 | 2048 | 4096 | 8192
      mask Callback debouce: waijung_intput_validation_callback('prescale');
      mask Display: disp('Button Pressed\n(Normal)');
  Debouce3 : Subsystem  TreatAsAtomicUnit=on  mask{mode=Single Pulse, prescale=4, debouce=3}
      mask prompts: prescale "Prescale (Debouce count)"; debouce "Debouce value"
      settings: RTWFcnNameOpts=Use subsystem name  RTWFileNameOpts=Use function name
      mask TypeOptions mode: Normal | Single Pulse | Toggle Latch
      mask Callback mode: waijung_intput_validation_callback('mode');
      mask TypeOptions prescale: 4 | 8 | 16 | 32 | 64 | 128 | 256 | 512 | 1024 | 2048 | 4096 | 8192
      mask Callback debouce: waijung_intput_validation_callback('prescale');
      mask Display: disp('Button Pressed\n(Normal)');
  Generate Mode ID : Subsystem
  Logical Operator : Logic  Operator=OR  AllPortsSameDT=off  OutDataTypeStr=boolean
  Subsystem : Subsystem
  Adjust state : Outport
  wires:
  UP/1 -> Debouce2/1(In1)
  DOWN/1 -> Debouce3/1(In1)
  MODE/1 -> Debouce1/1(In1)
  Debouce1/1(Out1) -> Generate Mode ID/1(In1)
  Generate Mode ID/1(Out1) -> Adjust state/1, Subsystem/4(Adjust State)
  Debouce3/1(Out1) -> Logical Operator/2, Subsystem/2(Down)
  Debouce2/1(Out1) -> Logical Operator/1, Subsystem/1(Up)
  Logical Operator/1 -> Subsystem/Enable
  SlvAddr/1 -> Subsystem/3(SlvAddr)
